simulink model "scheme"  (R2020a)
settings: Solver=VariableStepAuto  StartTime=0.0  StopTime=10.0  RelTol=1e-3
settings Model: Creator=ILIA  LastModifiedBy=ILIA

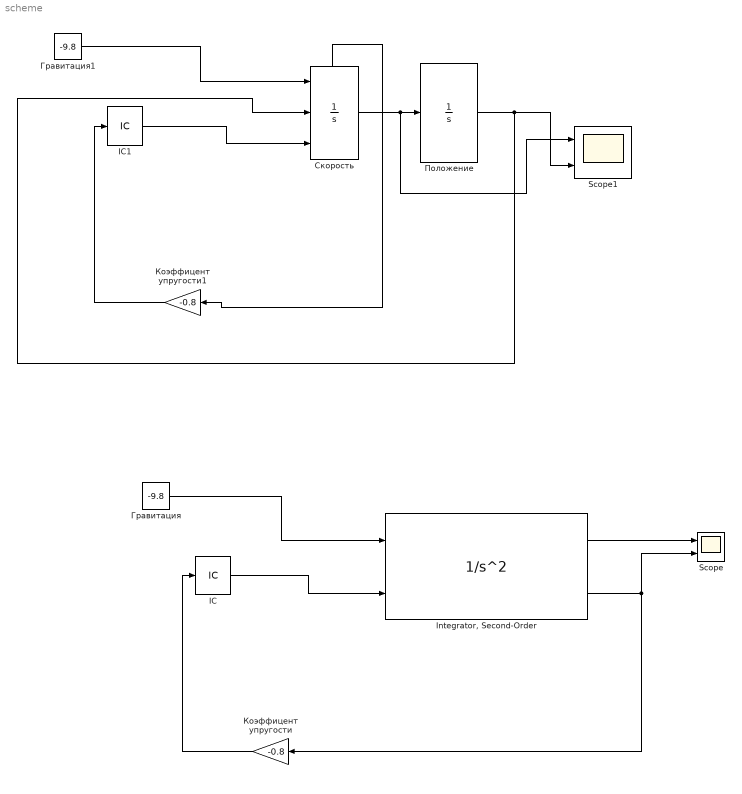
== system scheme ==
  IC : InitialCondition  Value=15
  IC1 : InitialCondition  Value=15
  "Integrator, Second-Order" : SecondOrderIntegrator  ICX=10  LimitX=on  LowerLimitX=0  ICSourceDXDT=external  ICDXDT=10  LowerLimitDXDT=0  ReinitDXDTwhenXreachesSaturation=on
  Scope : Scope  NumInputPorts=2
  Scope1 : Scope  NumInputPorts=2
  Гравитация : Constant  Value=-9.8
  Гравитация1 : Constant  Value=-9.8
  Коэффицент упругости : Gain  Gain=-0.8
  Коэффицент упругости1 : Gain  Gain=-0.8
  Положение : Integrator  InitialCondition=10  LimitOutput=on  LowerSaturationLimit=0
  Скорость : Integrator  ExternalReset=falling  InitialConditionSource=external  ShowStatePort=on
  wires:
  Коэффицент упругости/1 -> IC/1
  "Integrator, Second-Order"/1 -> Scope/1
  "Integrator, Second-Order"/2 -> Scope/2, Коэффицент упругости/1
  IC/1 -> "Integrator, Second-Order"/2
  Гравитация/1 -> "Integrator, Second-Order"/1
  Коэффицент упругости1/1 -> IC1/1
  IC1/1 -> Скорость/3
  Скорость/1 -> Scope1/1, Положение/1
  Скорость/State -> Коэффицент упругости1/1
  Положение/1 -> Скорость/2, Scope1/2
  Гравитация1/1 -> Скорость/1
